simulink model "Test_MotionSM_Motor"  (R2017b)
settings: Solver=FixedStepAuto  StartTime=0.0  StopTime=1000  FixedStep=0.001  RelTol=1e-3
settings Model: Creator=张紫薇  LastModifiedBy=张紫薇

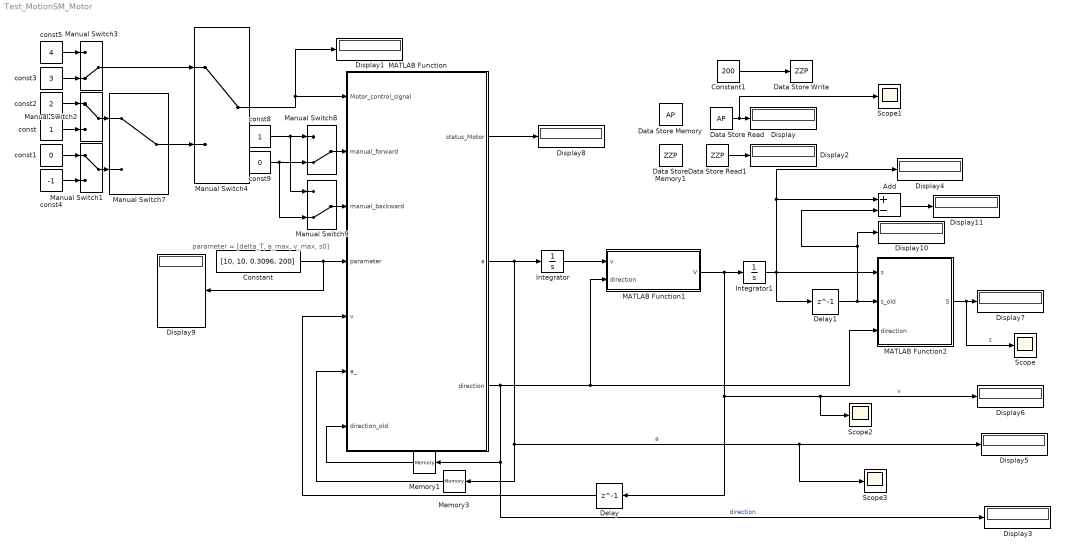
== system Test_MotionSM_Motor ==
  note: parameter = [delta_T, a_max, v_max, s0]
  Add : Sum  Inputs=+-
  Constant : Constant  Value=[10, 10, 0.3096, 200]
  Constant1 : Constant  Value=200
  Data Store Memory : DataStoreMemory  DataStoreName=AP  ReadBeforeWriteMsg=warning  WriteAfterWriteMsg=warning  WriteAfterReadMsg=warning  ShowAdditionalParam=off  OutDataTypeStr=double  Dimensions=1
  Data Store Memory1 : DataStoreMemory  DataStoreName=ZZP  ReadBeforeWriteMsg=warning  WriteAfterWriteMsg=warning  WriteAfterReadMsg=warning  ShowAdditionalParam=off  OutDataTypeStr=double  Dimensions=1
  Data Store Read : DataStoreRead  DataStoreName=AP
  Data Store Read1 : DataStoreRead  DataStoreName=ZZP
  Data Store Write : DataStoreWrite  DataStoreName=ZZP
  Delay : Delay  DelayLength=1
  Delay1 : Delay  DelayLength=1
  Display{,1..11} (12 alike) : Display
      Display5 settings: Format=decimal (Stored Integer)
      Display6 settings: Format=decimal (Stored Integer)
      Display7 settings: Format=decimal (Stored Integer)
  Integrator : Integrator
  Integrator1 : Integrator
  MATLAB Function : MATLAB Function  TreatAsAtomicUnit=on
  MATLAB Function1 : MATLAB Function  TreatAsAtomicUnit=on
  MATLAB Function2 : MATLAB Function  TreatAsAtomicUnit=on
  Manual Switch{1..2,4,7} (4 alike) : ManualSwitch
  Manual Switch3 : ManualSwitch  CurrentSetting=0
  Manual Switch8 : ManualSwitch  CurrentSetting=0
  Manual Switch9 : ManualSwitch  CurrentSetting=0
  Memory1 : Memory
  Memory3 : Memory
  Scope{,1..3} (4 alike) : Scope
  const : Constant  OutDataTypeStr=double
  const1 : Constant  Value=0  OutDataTypeStr=double
  const2 : Constant  Value=2  OutDataTypeStr=double
  const3 : Constant  Value=3  OutDataTypeStr=double
  const4 : Constant  Value=-1  OutDataTypeStr=double
  const5 : Constant  Value=4  OutDataTypeStr=double
  const8 : Constant  OutDataTypeStr=boolean
  const9 : Constant  Value=0  OutDataTypeStr=boolean
  wires:
  const4/1 -> Manual Switch1/2
  const1/1 -> Manual Switch1/1
  const2/1 -> Manual Switch2/1
  const/1 -> Manual Switch2/2
  const5/1 -> Manual Switch3/1
  const3/1 -> Manual Switch3/2
  Manual Switch2/1 -> Manual Switch7/1
  Manual Switch1/1 -> Manual Switch7/2
  Manual Switch3/1 -> Manual Switch4/1
  Manual Switch7/1 -> Manual Switch4/2
  Memory3/1 -> MATLAB Function/6(a_)
  MATLAB Function/3(direction) -> Display3/1, Memory1/1, MATLAB Function1/2(direction), MATLAB Function2/3(direction)  "direction"
  MATLAB Function2/1(S) -> Scope/1, Display7/1  "s"
  Delay1/1 -> Add/2, Display10/1, MATLAB Function2/2(s_old)
  MATLAB Function1/1(V) -> Integrator1/1, Delay/1, Scope2/1, Display6/1  "v"
  MATLAB Function/2(a) -> Integrator/1, Scope3/1, Display5/1, Memory3/1  "a"
  Integrator1/1 -> Delay1/1, Display4/1, Add/1, MATLAB Function2/1(s)
  Manual Switch4/1 -> Display1/1, MATLAB Function/1(Motor_control_signal)
  Integrator/1 -> MATLAB Function1/1(v)
  MATLAB Function/1(status_Motor) -> Display8/1
  Memory1/1 -> MATLAB Function/7(direction_old)
  Delay/1 -> MATLAB Function/5(v)
  Constant/1 -> MATLAB Function/4(parameter), Display9/1
  const8/1 -> Manual Switch9/1, Manual Switch8/1
  Manual Switch8/1 -> MATLAB Function/2(manual_forward)
  Manual Switch9/1 -> MATLAB Function/3(manual_backward)
  const9/1 -> Manual Switch9/2, Manual Switch8/2
  Data Store Read/1 -> Scope1/1, Display/1
  Data Store Read1/1 -> Display2/1
  Constant1/1 -> Data Store Write/1
  Add/1 -> Display11/1

== matlab function Test_MotionSM_Motor/MATLAB Function ==
  settings: updateMethod=DISCRETE
  data: status_Motor output boolean size=1; Motor_control_signal input double size=1; manual_forward input boolean size=1; manual_backward input boolean size=1; parameter input double size=4; v input double size=1; a_ input; direction_old input; a output double size=1; direction output double size=1; AP data_store_memory; ZZP data_store_memory
function [status_Motor, a, direction]= Motor(Motor_control_signal, manual_forward, manual_backward, parameter, v, a_, direction_old)

%delta_T = parameter(1);
a_max = parameter(2);
v_max = parameter(3);
s0 = parameter(4);
direction = 0;
a = 0;

s_a = 0.5*v_max*v_max/a_max;
a_bremsen = 200;

global AP
global ZZP

switch Motor_control_signal
    case -1                 %Error
        if v > 0
            a = -a_bremsen;
            direction = 1;
        elseif v < 0
            a = a_bremsen;
            direction = -1;
        else
            a = 0;
            direction = 0;
        end
        
    case 0                  %Off
        if v > 0
            a = -a_max;
            direction = 1;
        elseif v < 0
            a = a_max;
            direction = -1;
        else
            a = 0;
            direction = 0;
        end
        
    case 1                  %Init
        if AP > 0
            direction = -1;
            if (AP > abs(s_a)) && (v > (-v_max/10)) && (v < 0)
                a = -a_max;
            elseif (AP > abs(s_a)) && (v <= (-v_max/10)) || (v >= 0)
                a = 0;
            elseif (AP <= abs(s_a)) && (AP > 0) && (v < 0)
                a = a_max;
            else
                a = 0;
                AP = 0;
            end
        end
        
    case 2                  %Stop
        if v > 0
            a = -a_max;
            direction = 1;
        elseif v < 0
            a = a_max;
            direction = -1;
        else
            a = 0;
            direction = 0;
        end
        
    case 3                  %run
        direction = s0;
        if (s0 > 0)   %forward
            %v_control(2) = s0;
            if ((ZZP - AP) > s_a) && (v < v_max)
                a = a_max;
            elseif ((ZZP - AP) <= s_a) && (ZZP > AP) && (v > 0)
                a = -a_max;
            else
                a = 0;
            end
        end
        if (s0 < 0)    %backward
            if ((ZZP - AP) < -s_a) && (v > -v_max)
                a = -a_max;
            elseif ((ZZP - AP) >= -s_a) && (ZZP < AP) && (v < 0)
                a = a_max;
            else
                a = 0;
            end
        end
        
    case 4                  %Manual_control
        if manual_forward
            direction = 1;
            if v < v_max
                a = a_max;
            else
                a = 0;
            end
        end
        if manual_backward
            direction = -1;
            if v > -v_max
                a = -a_max;
            else
                a = 0;
            end
        end
        if ((~manual_forward) && (~manual_backward))
            if v > 0 && (direction_old == 1)
                a = -a_max;
            elseif v < 0 && (direction_old == -1)
                a = a_max;
            else
                a = 0;
            end
        end 
end

%AP = AP + s - s_old;
%s_new = s;

%status_Motor: false...Stopped, true...Running
if (a == 0) && (v == 0)
    status_Motor = false;
else
    status_Motor = true;
end

end

== matlab function Test_MotionSM_Motor/MATLAB Function1 ==
  settings: updateMethod=DISCRETE
  data: V output; v input; direction input double size=1; AP data_store_memory; ZZP data_store_memory
function V = v_conrol(v, direction)
global AP
global ZZP

if direction > 0
    if v < 0 || (AP >= ZZP)
        V = 0;
    else
        V = v;
    end
elseif direction < 0
    if v > 0 || (AP <= ZZP)
        V = 0;
    else
        V = v;
    end
else
    V = 0;
end

end

== matlab function Test_MotionSM_Motor/MATLAB Function2 ==
  settings: updateMethod=DISCRETE
  data: s input; s_old input; S output; direction input double size=1; AP data_store_memory; ZZP data_store_memory
function S = s_control(s, s_old, direction)

global AP
global ZZP

if direction > 0
    if (AP + s - s_old) < ZZP
        S = s;
        AP = AP + s - s_old;
    else
        S = s_old;
        AP = ZZP;
    end

elseif direction < 0
    if (AP + s - s_old) > ZZP
        S = s;
        AP = AP + s - s_old;
    else
        S = s_old;
        AP = ZZP;
    end
else
    S = s_old;
end

end
